simulink model "sampleModel227"  (R2021b)
settings: Solver=VariableStepAuto  StartTime=0.0  StopTime=10.0  RelTol=1e-3
undefined symbols (not defined in the file or in its folder): DiscIntNeverNeededParam
libraries: simulink x11, slpidlib x1
settings Model: Creator=user  LastModifiedBy=user

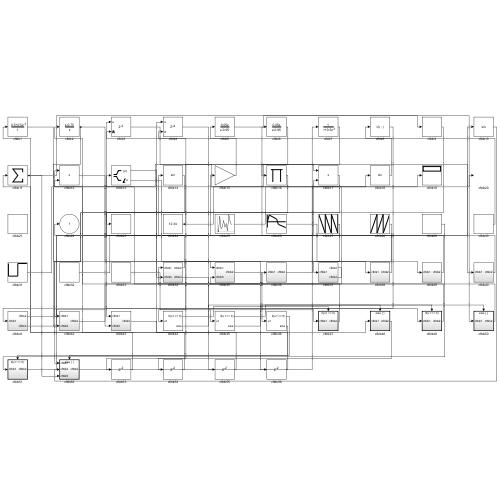
[thumbnail: Simulink's stored preview of the top-level diagram]
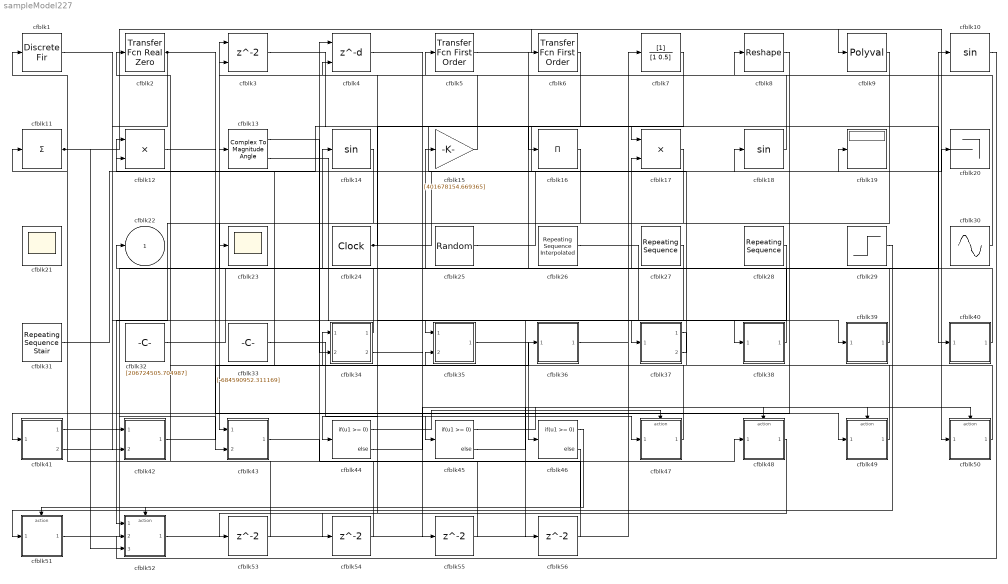
== system sampleModel227 ==
  cfblk1 : DiscreteFir  SampleTime=1
  cfblk10 : Trigonometry
  cfblk11 : Sum  Inputs=+
  cfblk12 : Product  Inputs=**
  cfblk13 : ComplexToMagnitudeAngle
  cfblk14 : Trigonometry
  cfblk15 : Gain  Gain=[401678154.669365]
  cfblk16 : Product  Inputs=*
  cfblk17 : Product  Inputs=**
  cfblk18 : Trigonometry
  cfblk19 : Display
  cfblk2 : simulink/Discrete/Transfer Fcn Real Zero  ZeroZ=0.75  ICPrevInput=0.0  DoSatur=off
      settings: SourceProductBaseCode=SL
  cfblk20 : Terminator
  cfblk21 : Scope
      settings: Floating=on
  cfblk23 : Scope
  cfblk24 : DigitalClock
  cfblk25 : UniformRandomNumber  Minimum=[-9424979121.208391]  Maximum=[4576921704.532799]  Seed=[56371023.000000]  SampleTime=0.1
  cfblk26 : simulink/Sources/Repeating Sequence Interpolated  OutValues=[-68559920.033073, 851527944.369656, 309275423.802970, -325161568.673075, -741238021.355165]  TimeValues=[0 0.1 0.5 0.6 1].'  LookUpMeth=Use Input Above  tsamp=0.01  OutMin=[]  OutMax=[]  OutDataTypeStr=double  OutputDataTypeScalingMode=double  OutDataType=fixdt(0,8)  OutScaling=2^-10
  cfblk27 : simulink/Sources/Repeating Sequence  rep_seq_t=[0 2]  rep_seq_y=[762800476.292960, -842250220.652404]
  cfblk28 : simulink/Sources/Repeating Sequence  rep_seq_t=[0 2]  rep_seq_y=[29823164.683198, 536430253.252818]
  cfblk29 : Step  Time=[37.000000]  Before=[111936378.065930]  After=[-634457052.127596]  SampleTime=0
  cfblk3 : Delay  ShowEnablePort=on  SampleTime=1
      settings: InputPortMap=u0,e6
  cfblk30 : Sin  Amplitude=[793889132.243178]  Bias=[419481654.251079]  SampleTime=0
  cfblk31 : simulink/Sources/Repeating Sequence Stair  OutValues=[309216023.549124, 880544981.325996]  tsamp=-1  OutMin=[]  OutMax=[]  OutDataTypeStr=double  OutputDataTypeScalingMode=double  OutDataType=fixdt(0,8)  ConRadixGroup=Best Precision: Vector-wise  OutScaling=2^-12
  cfblk32 : Constant  Value=[206724505.704987]  SampleTime=1
  cfblk33 : Constant  Value=[-684590952.311169]  SampleTime=1
  cfblk34 : Subsystem
  cfblk35 : Subsystem
  cfblk36 : Subsystem
  cfblk37 : Subsystem
  cfblk38 : Subsystem
  cfblk39 : Subsystem
  cfblk4 : Delay  DelayLengthSource=Input port  SampleTime=1
      settings: InputPortMap=u0,p1
  cfblk40 : Subsystem
  cfblk41 : Subsystem
  cfblk42 : Subsystem
  cfblk43 : Subsystem
  cfblk44 : If  IfExpression=u1 >= 0  SampleTime=1
  cfblk45 : If  IfExpression=u1 >= 0  SampleTime=1
  cfblk46 : If  IfExpression=u1 >= 0  SampleTime=1
  cfblk47 : Subsystem  TreatAsAtomicUnit=on
  cfblk48 : Subsystem  TreatAsAtomicUnit=on
  cfblk49 : Subsystem  TreatAsAtomicUnit=on
  cfblk5 : simulink/Discrete/Transfer Fcn First Order  PoleZ=0.95  ICPrevOutput=0.0  DoSatur=off
  cfblk50 : Subsystem  TreatAsAtomicUnit=on
  cfblk51 : Subsystem  TreatAsAtomicUnit=on
  cfblk52 : Subsystem  TreatAsAtomicUnit=on
  cfblk{53..56} (4 alike) : Delay  SampleTime=1
  cfblk6 : simulink/Discrete/Transfer Fcn First Order  PoleZ=0.95  ICPrevOutput=0.0  DoSatur=off
  cfblk7 : DiscreteFilter  SampleTime=1
  cfblk8 : Reshape
  cfblk9 : Polyval  Coefs=[ +2.081618890e-019, -1.441693666e-014, +4.719686976e-010, -8.536869453e-006, +1.621573104e-001, -8.087801117e+001 ]
  cfblk22 : Outport
  wires:
  cfblk18/1 -> cfblk3/1
  cfblk8/1 -> cfblk41/1(cfblk1)
  cfblk49/1(cfblk2) -> cfblk34/1(cfblk1)
  cfblk35/1(cfblk2) -> cfblk46/1
  cfblk34/1(cfblk2) -> cfblk22/1
  cfblk16/1 -> cfblk43/1(cfblk1)
  cfblk28/1 -> cfblk37/1(cfblk1)
  cfblk11/1 -> cfblk50/1(cfblk1), cfblk52/3(cfblk5)
  cfblk29/1 -> cfblk51/1(cfblk1)
  cfblk39/1(cfblk2) -> cfblk14/1
  cfblk30/1 -> cfblk8/1
  cfblk25/1 -> cfblk18/1
  cfblk15/1 -> cfblk5/1
  cfblk31/1 -> cfblk17/1
  cfblk27/1 -> cfblk44/1
  cfblk26/1 -> cfblk39/1(cfblk1)
  cfblk5/1 -> cfblk9/1
  cfblk33/1 -> cfblk45/1
  cfblk24/1 -> cfblk20/1, cfblk4/2
  cfblk43/1(cfblk2) -> cfblk48/1(cfblk1)
  cfblk42/1(cfblk2) -> cfblk36/1(cfblk1)
  cfblk52/1(cfblk2) -> cfblk7/1
  cfblk3/1 -> cfblk40/1(cfblk1)
  cfblk38/1(cfblk2) -> cfblk3/2
  cfblk41/1(cfblk2) -> cfblk43/2(cfblk5)
  cfblk2/1 -> cfblk38/1(cfblk1), cfblk42/2(cfblk5)
  cfblk41/2(cfblk3) -> cfblk10/1
  cfblk1/1 -> cfblk35/1(cfblk1)
  cfblk51/1(cfblk2) -> cfblk15/1
  cfblk13/1 -> cfblk34/2(cfblk3)
  cfblk32/1 -> cfblk17/2
  cfblk36/1(cfblk2) -> cfblk19/1
  cfblk47/1(cfblk2) -> cfblk12/1
  cfblk9/1 -> cfblk23/1
  cfblk4/1 -> cfblk47/1(cfblk1)
  cfblk50/1(cfblk2) -> cfblk13/1
  cfblk17/1 -> cfblk52/1(cfblk1)
  cfblk10/1 -> cfblk52/2(cfblk4)
  cfblk40/1(cfblk2) -> cfblk6/1
  cfblk37/1(cfblk2) -> cfblk35/2(cfblk5)
  cfblk14/1 -> cfblk42/1(cfblk1)
  cfblk37/2(cfblk4) -> cfblk12/2
  cfblk7/1 -> cfblk16/1
  cfblk12/1 -> cfblk49/1(cfblk1)
  cfblk44/1 -> cfblk47/Action
  cfblk44/2 -> cfblk48/Action
  cfblk45/1 -> cfblk49/Action
  cfblk45/2 -> cfblk50/Action
  cfblk46/1 -> cfblk51/Action
  cfblk46/2 -> cfblk52/Action
  cfblk48/1(cfblk2) -> cfblk53/1
  cfblk53/1 -> cfblk1/1
  cfblk6/1 -> cfblk54/1
  cfblk54/1 -> cfblk2/1
  cfblk34/2(cfblk4) -> cfblk55/1
  cfblk55/1 -> cfblk4/1
  cfblk13/2 -> cfblk56/1
  cfblk56/1 -> cfblk11/1

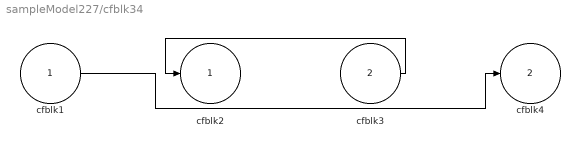
== system sampleModel227/cfblk34 ==
  cfblk1 : Inport
  cfblk3 : Inport  Port=2
  cfblk2 : Outport
  cfblk4 : Outport  Port=2
  wires:
  cfblk3/1 -> cfblk2/1
  cfblk1/1 -> cfblk4/1

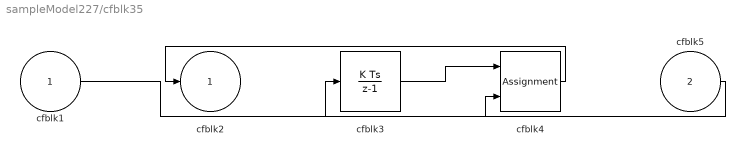
== system sampleModel227/cfblk35 ==
  cfblk1 : Inport
  cfblk5 : Inport  Port=2
  cfblk3 : DiscreteIntegrator  ICPrevOutput=DiscIntNeverNeededParam  ICPrevScaledInput=DiscIntNeverNeededParam
  cfblk4 : Assignment  DiagnosticForDimensions=Warning  IndexOptions=Index vector (dialog)  Indices=1  OutputSizes=1
  cfblk2 : Outport
  wires:
  cfblk4/1 -> cfblk2/1
  cfblk5/1 -> cfblk3/1
  cfblk3/1 -> cfblk4/1
  cfblk1/1 -> cfblk4/2

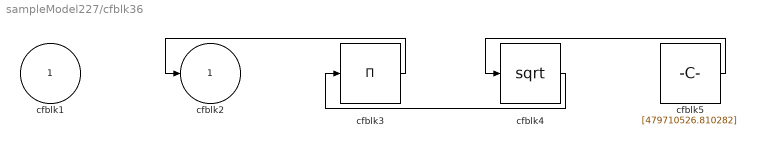
== system sampleModel227/cfblk36 ==
  cfblk1 : Inport
  cfblk3 : Product  Inputs=*
  cfblk4 : Sqrt  SaturateOnIntegerOverflow=on
  cfblk5 : Constant  Value=[479710526.810282]  SampleTime=1
  cfblk2 : Outport
  wires:
  cfblk5/1 -> cfblk4/1
  cfblk4/1 -> cfblk3/1
  cfblk3/1 -> cfblk2/1

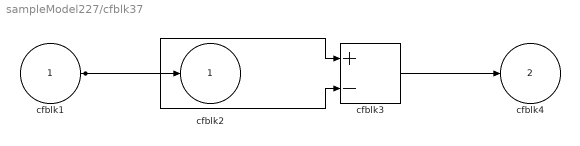
== system sampleModel227/cfblk37 ==
  cfblk1 : Inport
  cfblk3 : Sum  Inputs=+-
  cfblk2 : Outport
  cfblk4 : Outport  Port=2
  wires:
  cfblk3/1 -> cfblk4/1
  cfblk1/1 -> cfblk2/1, cfblk3/1, cfblk3/2

== system sampleModel227/cfblk38 ==
  cfblk1 : Inport
  cfblk3 : Squeeze
  cfblk4 : Constant  Value=[-158322974.185996]  SampleTime=1
  cfblk2 : Outport
  wires:
  cfblk1/1 -> cfblk2/1
  cfblk4/1 -> cfblk3/1

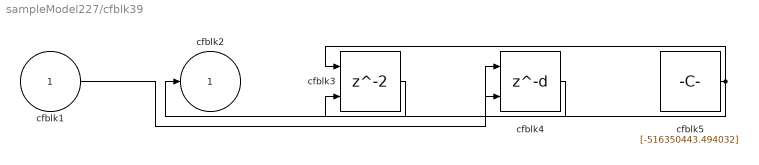
== system sampleModel227/cfblk39 ==
  cfblk1 : Inport
  cfblk3 : Delay  ShowEnablePort=on  SampleTime=1
      settings: InputPortMap=u0,e6
  cfblk4 : Delay  DelayLengthSource=Input port  SampleTime=1
      settings: InputPortMap=u0,p1
  cfblk5 : Constant  Value=[-516350443.494032]  SampleTime=1
  cfblk2 : Outport
  wires:
  cfblk5/1 -> cfblk3/1, cfblk4/2
  cfblk3/1 -> cfblk2/1
  cfblk1/1 -> cfblk4/1
  cfblk4/1 -> cfblk3/2

== system sampleModel227/cfblk40 ==
  cfblk1 : Inport
  cfblk3 : Constant  Value=[-947565933.944476]  SampleTime=1
  cfblk4 : Constant  Value=[-979831532.050449]  SampleTime=1
  cfblk2 : Outport
  wires:
  cfblk3/1 -> cfblk2/1

== system sampleModel227/cfblk41 ==
  cfblk1 : Inport
  cfblk2 : Outport
  cfblk3 : Outport  Port=2
  wires:
  cfblk1/1 -> cfblk3/1, cfblk2/1

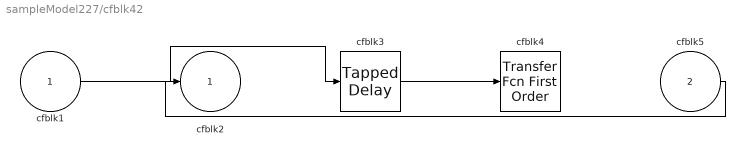
== system sampleModel227/cfblk42 ==
  cfblk1 : Inport
  cfblk5 : Inport  Port=2
  cfblk3 : simulink/Discrete/Tapped Delay  vinit=0.0  samptime=-1  NumDelays=1  DelayOrder=Oldest  includeCurrent=off
  cfblk4 : simulink/Discrete/Transfer Fcn First Order  PoleZ=0.95  ICPrevOutput=0.0  DoSatur=off
  cfblk2 : Outport
  wires:
  cfblk1/1 -> cfblk3/1
  cfblk5/1 -> cfblk2/1
  cfblk3/1 -> cfblk4/1

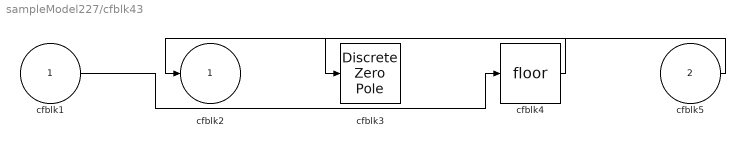
== system sampleModel227/cfblk43 ==
  cfblk1 : Inport
  cfblk5 : Inport  Port=2
  cfblk3 : DiscreteZeroPole  Poles=[0 0.5]  Gain=1
  cfblk4 : Rounding
  cfblk2 : Outport
  wires:
  cfblk5/1 -> cfblk2/1
  cfblk1/1 -> cfblk4/1
  cfblk4/1 -> cfblk3/1

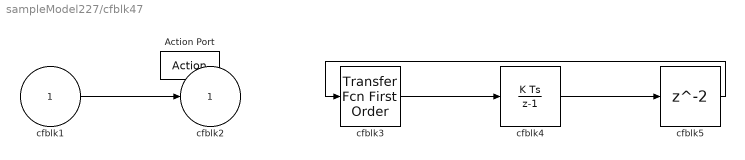
== system sampleModel227/cfblk47 ==
  cfblk1 : Inport
  Action Port : ActionPort  ActionPortLabel=if(u1 >= 0)
  cfblk3 : simulink/Discrete/Transfer Fcn First Order  PoleZ=0.95  ICPrevOutput=0.0  DoSatur=off
  cfblk4 : DiscreteIntegrator  SampleTime=-1  ICPrevOutput=DiscIntNeverNeededParam  ICPrevScaledInput=DiscIntNeverNeededParam
  cfblk5 : Delay
  cfblk2 : Outport
  wires:
  cfblk3/1 -> cfblk4/1
  cfblk1/1 -> cfblk2/1
  cfblk4/1 -> cfblk5/1
  cfblk5/1 -> cfblk3/1

== system sampleModel227/cfblk48 ==
  cfblk1 : Inport
  Action Port : ActionPort  ActionPortLabel=else
  cfblk3 : simulink/Discrete/Difference  ICPrevInput=0.0  OutMin=[]  OutMax=[]  OutDataTypeStr=Inherit: Inherit via back propagation  OutDataType=fixdt(1, 16)  OutScaling=2^-10  DoSatur=off
  cfblk2 : Outport
  wires:
  cfblk1/1 -> cfblk3/1
  cfblk3/1 -> cfblk2/1

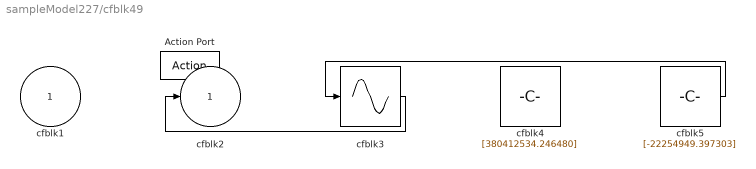
== system sampleModel227/cfblk49 ==
  cfblk1 : Inport
  Action Port : ActionPort  ActionPortLabel=if(u1 >= 0)
  cfblk3 : Sin  TimeSource=Use external signal  SampleTime=0
  cfblk4 : Constant  Value=[380412534.246480]  SampleTime=1
  cfblk5 : Constant  Value=[-22254949.397303]  SampleTime=1
  cfblk2 : Outport
  wires:
  cfblk5/1 -> cfblk3/1
  cfblk3/1 -> cfblk2/1

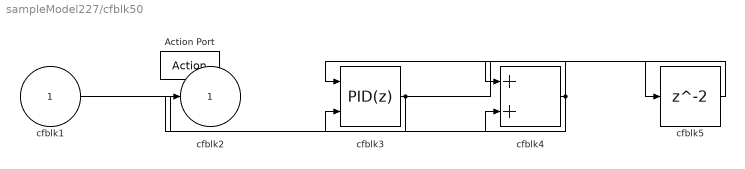
== system sampleModel227/cfblk50 ==
  cfblk1 : Inport
  Action Port : ActionPort  ActionPortLabel=else
  cfblk3 : slpidlib/PID Controller (2DOF)  Controller=PID  Form=Parallel  TimeDomain=Discrete-time  UseExternalTs=off  SampleTime=-1  IntegratorMethod=Forward Euler  FilterMethod=Forward Euler  ControllerParametersSource=internal  P=1  I=1  D=0  UseFilter=on  N=100  b=1  c=1  TunerSelectOption=Transfer Function Based (PID Tuner App)  InitialConditionSource=internal  InitialConditionForIntegrator=0  InitialConditionForFilter=0  DifferentiatorICPrevScaledInput=0  ExternalReset=none  TrackingMode=off  Kt=1  LimitOutput=off  SatLimitsSource=internal  UpperSaturationLimit=inf  LowerSaturationLimit=-inf  LinearizeAsGain=off  AntiWindupMode=none  Kb=1  POutMin=[]  POutMax=[]  IOutMin=[]  IOutMax=[]  DOutMin=[]  DOutMax=[]  NOutMin=[]  NOutMax=[]  bOutMin=[]  bOutMax=[]  cOutMin=[]  cOutMax=[]  SumOutMin=[]  SumOutMax=[]  SaturationOutMin=[]  SaturationOutMax=[]  PParamMin=[]  PParamMax=[]  IParamMin=[]  IParamMax=[]  DParamMin=[]  DParamMax=[]  NParamMin=[]  NParamMax=[]  bParamMin=[]  bParamMax=[]  cParamMin=[]  cParamMax=[]  KbParamMin=[]  KbParamMax=[]  KtParamMin=[]  KtParamMax=[]  KbOutMin=[]  KbOutMax=[]  KtOutMin=[]  KtOutMax=[]  IntegratorOutMin=[]  IntegratorOutMax=[]  FilterOutMin=[]  FilterOutMax=[]  SumI1OutMin=[]  SumI1OutMax=[]  SumI2OutMin=[]  SumI2OutMax=[]  SumI3OutMin=[]  SumI3OutMax=[]  SumI4OutMin=[]  SumI4OutMax=[]  SumDOutMin=[]  SumDOutMax=[]  Sum1OutMin=[]  Sum1OutMax=[]  Sum2OutMin=[]  Sum2OutMax=[]  Sum3OutMin=[]  Sum3OutMax=[]  DifferentiatorOutMin=[]  DifferentiatorOutMax=[]  FilterDiffOutCoefMin=[]  FilterDiffOutCoefMax=[]  ReciprocalOutMin=[]  ReciprocalOutMax=[]  SumDenOutMin=[]  SumDenOutMax=[]  SumNumOutMin=[]  SumNumOutMax=[]  DivideOutMin=[]  DivideOutMax=[]  UdiffTsProdOutMin=[]  UdiffTsProdOutMax=[]  NTsProdOutMin=[]  NTsProdOutMax=[]  UintegralTsProdOutMin=[]  UintegralTsProdOutMax=[]  UngainTsProdOutMin=[]  UngainTsProdOutMax=[]  IntegratorContinuousStateAttributes=''  IntegratorStateMustResolveToSignalObject=off  IntegratorRTWStateStorageClass=Auto  FilterContinuousStateAttributes=''  FilterStateMustResolveToSignalObject=off  FilterRTWStateStorageClass=Auto  ParallelPVariant=InternalParameters  IdealPVariant=Disabled  IVariant=InternalParameters  DVariant=InternalParameters  bVariant=InternalParameters  cVariant=InternalParameters  IntegratorVariant=Discrete  SatVariant=Disabled  AWVariant=Passthrough  PCopyVariant=Disabled  TRVariant=Disabled  FdbkBlocksVariant=Forward  IdealPFdbkVariant=Disabled  SatFdbkVariant=Disabled  DerivativeFilterVariant=ForwardEulerFilter  NVariant=InternalParameters  NCopyVariant=Disabled  FilterICVariant=InternalICsFilter  IntegratorICVariant=InternalICs  ExternalResetVariant=Disabled  TRSumVariant=Passthrough  SumFdbkVariant=Disabled  SumVariant=Sum_PID  TsampFilterVariant=InternalTs  TsampNgainVariant=Passthrough  TsampIntegralVariant=Passthrough  ExternalSaturationOutDataTypeStr=Inherit: Same as second input
      settings: SourceProductBaseCode=SL
  cfblk4 : Sum
  cfblk5 : Delay
  cfblk2 : Outport
  wires:
  cfblk4/1 -> cfblk3/1, cfblk3/2
  cfblk3/1 -> cfblk2/1, cfblk5/1
  cfblk1/1 -> cfblk4/2
  cfblk5/1 -> cfblk4/1

== system sampleModel227/cfblk51 ==
  cfblk1 : Inport
  Action Port : ActionPort  ActionPortLabel=if(u1 >= 0)
  cfblk3 : Squeeze
  cfblk2 : Outport
  wires:
  cfblk3/1 -> cfblk2/1
  cfblk1/1 -> cfblk3/1

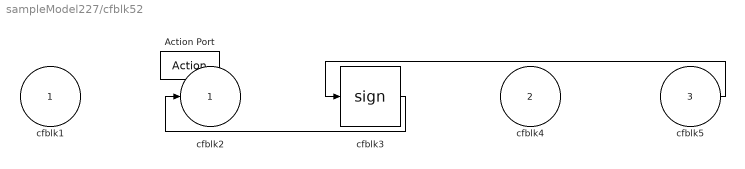
== system sampleModel227/cfblk52 ==
  cfblk1 : Inport
  cfblk4 : Inport  Port=2
  cfblk5 : Inport  Port=3
  Action Port : ActionPort  ActionPortLabel=else
  cfblk3 : Signum
  cfblk2 : Outport
  wires:
  cfblk3/1 -> cfblk2/1
  cfblk5/1 -> cfblk3/1
